simulink model "Acq_track"  (R2019b)
settings: Solver=VariableStepAuto  StartTime=0.0  StopTime=1  FixedStep=1/fs  RelTol=1e-3  EnableMultiTasking=on
values from neighbouring files (symbols this model uses):
  freq_vector = 2*pi*[(fc - 10e3):1e3:(fc+10e3)]    [config.m]
  fs = 16367600    [config.m]    (also in trackingCode.m)
  Len = ceil(ms*fs/1000)    [config.m]    (also in trackingCode.m = ceil((codeLength - remCodePhase)/(ca_freq/fs)))
  switch_time = 8*Len/fs    [config.m]
libraries: dspsigops x7, commfilt2 x6, dspstat3 x2, commseqgen3 x2, dspsrcs4 x1, simulink x1, simulink_extras x1
settings Model: Creator=nishantmittal  LastModifiedBy=sanke
settings SolverCC: AutoInsertRateTranBlk=on
settings OptimizationCC: DefaultUnderspecifiedDataType=single
settings DebuggingCC: ParameterPrecisionLossMsg=none

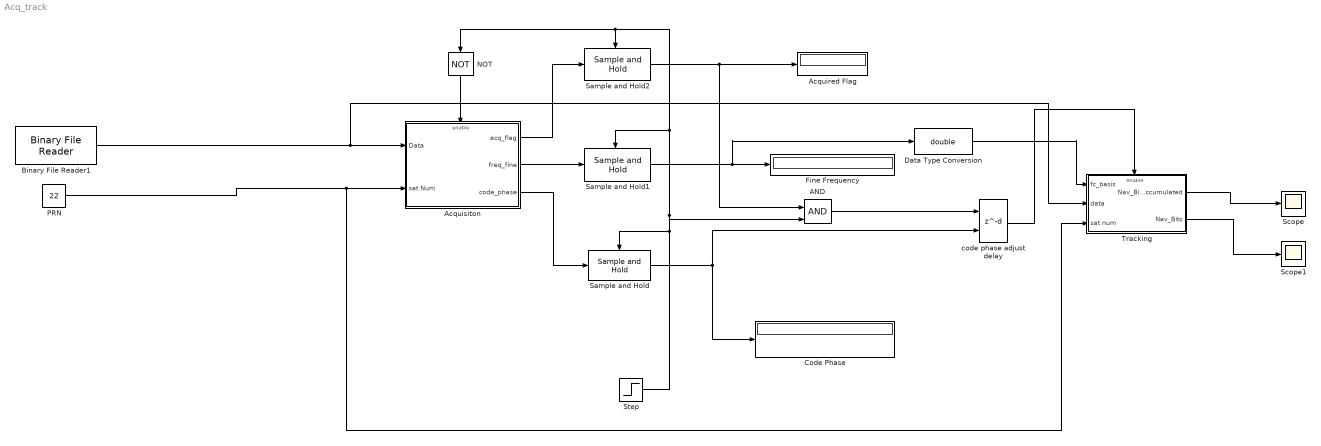
== system Acq_track ==
  AND : Logic  IconShape=distinctive  AllPortsSameDT=off  OutDataTypeStr=boolean
  Acquired Flag : Display
  Acquisiton : Subsystem
  Binary File Reader1 : dspsrcs4/Binary File Reader  Filename=/Users/nishantmittal/Documents/SURP/data/Acqisition/test/gioveAandB_short.bin  HeaderStructure=struct([])  DataType=int8  SamplesPerFrame=1  IsDataComplex=off  NumChannels=1  OutputEOF=off  SampleTime=1/fs  SimulateUsing=Code generation
      settings: SourceProductBaseCode=DS
  Code Phase : Display
  Data Type Conversion : DataTypeConversion  OutDataTypeStr=double
  Fine Frequency : Display
  NOT : Logic  Operator=NOT  IconShape=distinctive  AllPortsSameDT=off  OutDataTypeStr=boolean
  "PRN " : Constant  Value=22  OutDataTypeStr=single
  Sample and Hold : dspsigops/Sample and Hold  trig=Rising edge  initCond=0  latchinput=off
  Sample and Hold1 : dspsigops/Sample and Hold  trig=Rising edge  initCond=0  latchinput=off
  Sample and Hold2 : dspsigops/Sample and Hold  trig=Rising edge  initCond=0  latchinput=off
  Scope : Scope
  Scope1 : Scope
  Step : Step  Time=switch_time  SampleTime=1/fs
  Tracking : Subsystem
  code phase adjust delay : Delay  DelayLengthSource=Input port  DelayLength=1  DelayLengthUpperLimit=Len  InitialCondition=0  SampleTime=1/fs
      settings: InputPortMap=u0,p1
  wires:
  Binary File Reader1/1 -> Tracking/2(data), Acquisiton/1(Data)
  "PRN "/1 -> Tracking/3(sat num), Acquisiton/2(sat Num)
  Acquisiton/3(code_phase) -> Sample and Hold/1
  Sample and Hold/1 -> Code Phase/1, code phase adjust delay/2
  Acquisiton/2(freq_fine) -> Sample and Hold1/1
  Acquisiton/1(acq_flag) -> Sample and Hold2/1
  Step/1 -> AND/2, NOT/1, Sample and Hold2/Trigger, Sample and Hold1/Trigger, Sample and Hold/Trigger
  Tracking/1(Nav_Bits_Accumulated) -> Scope/1
  Sample and Hold1/1 -> Data Type Conversion/1, Fine Frequency/1
  AND/1 -> code phase adjust delay/1
  Sample and Hold2/1 -> AND/1, Acquired Flag/1
  NOT/1 -> Acquisiton/Enable
  code phase adjust delay/1 -> Tracking/Enable
  Data Type Conversion/1 -> Tracking/1(fc_basis)
  Tracking/2(Nav_Bits) -> Scope1/1

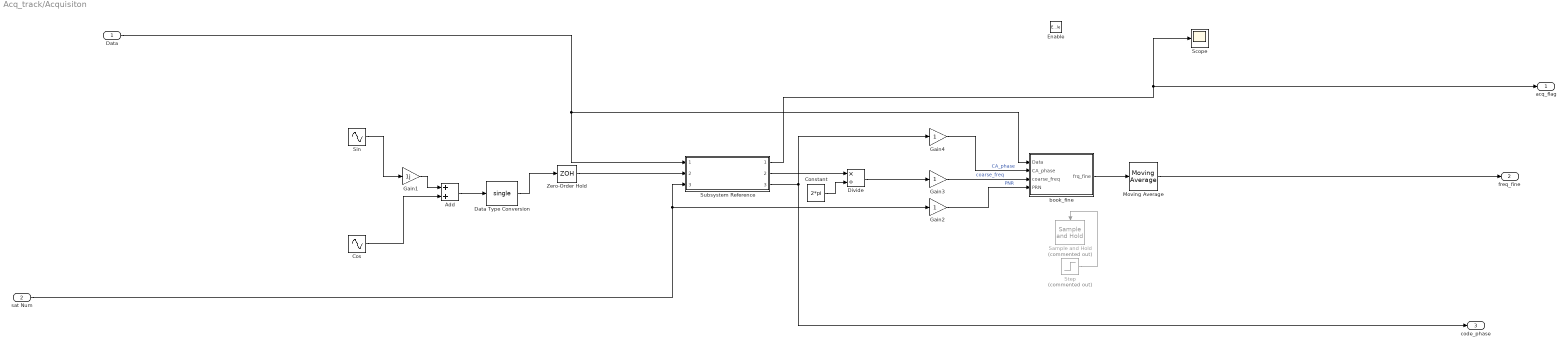
== system Acq_track/Acquisiton ==
  Data : Inport
  sat Num : Inport  Port=2
  Enable : EnablePort
  Add : Sum
  Constant : Constant  Value=2*pi  OutDataTypeStr=single
  Cos : Sin  Frequency=freq_vector  Phase=pi/2  SampleTime=1/fs
  Data Type Conversion : DataTypeConversion  OutDataTypeStr=single
  Divide : Product  Inputs=*/
  Gain1 : Gain  Gain=1j
  Gain2 : Gain
  Gain3 : Gain
  Gain4 : Gain  OutDataTypeStr=single
  Moving Average : dspstat3/Moving Average  Method=Sliding window  ForgettingFactorPort=off  SpecifyWindowLength=on  WindowLength=4  ForgettingFactor=0.9  SimulateUsing=Code generation
  Sample and Hold : dspsigops/Sample and Hold  Commented=on  trig=Rising edge  initCond=0  latchinput=off
  Scope : Scope
  "Sin " : Sin  Frequency=freq_vector  SampleTime=1/fs
  Step : Step  Commented=on  Time=0.00101  SampleTime=0
  Subsystem Reference : Subsystem  ReferencedSubsystem=acq_PNR
      settings: MinAlgLoopOccurrences=on
  Zero-Order Hold : ZeroOrderHold  SampleTime=1/fs
  book_fine : Subsystem
  acq_flag : Outport
  freq_fine : Outport  Port=2
  code_phase : Outport  Port=3
  wires:
  Moving Average/1 -> freq_fine/1
  Gain2/1 -> book_fine/4(PRN)  "PNR"
  Gain1/1 -> Add/1
  Subsystem Reference/2 -> Divide/1
  Data/1 -> book_fine/1(Data), Subsystem Reference/1
  Data Type Conversion/1 -> Zero-Order Hold/1
  "Sin "/1 -> Gain1/1
  Step/1 -> Sample and Hold/Trigger
  Gain4/1 -> book_fine/2(CA_phase)  "CA_phase"
  Add/1 -> Data Type Conversion/1
  Constant/1 -> Divide/2
  Cos/1 -> Add/2
  Gain3/1 -> book_fine/3(coarse_freq)  "coarse_freq"
  Subsystem Reference/1 -> acq_flag/1, Scope/1
  Divide/1 -> Gain3/1
  sat Num/1 -> Subsystem Reference/3, Gain2/1
  book_fine/1(frq_fine) -> Moving Average/1
  Zero-Order Hold/1 -> Subsystem Reference/2
  Subsystem Reference/3 -> code_phase/1, Gain4/1

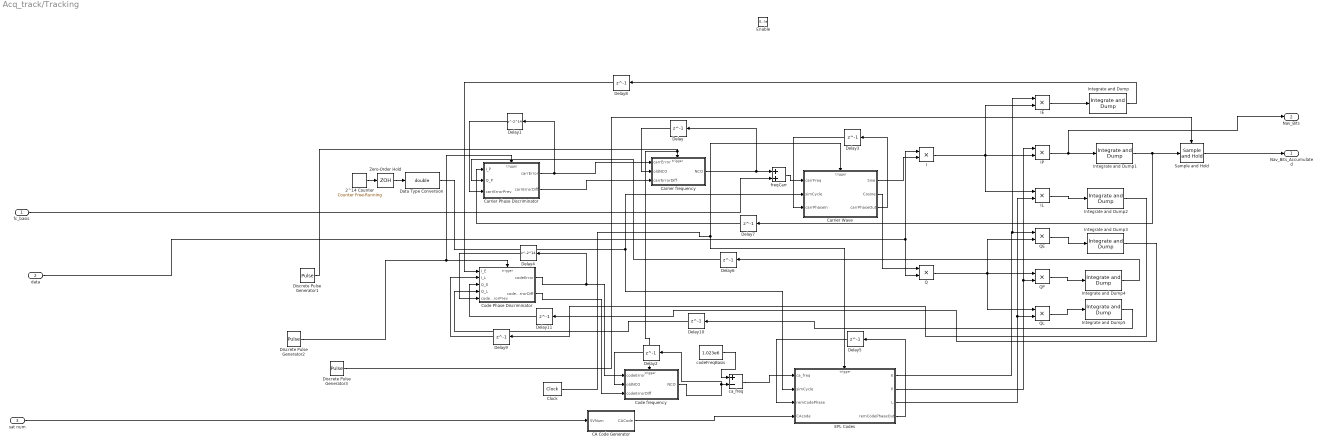
== system Acq_track/Tracking ==
  fc_basis : Inport
  data : Inport  Port=2
  sat num : Inport  Port=3
  Enable : EnablePort
  2^14 Counter : simulink/Sources/Counter Free-Running  NumBits=14  tsamp=1/fs
  CA Code Generator : Subsystem  TreatAsAtomicUnit=on
  Carrier Phase Discriminator : Subsystem  TreatAsAtomicUnit=on
  Carrier Wave : Subsystem  TreatAsAtomicUnit=on
  Carrier frequency : Subsystem  TreatAsAtomicUnit=on
  Clock : simulink_extras/Flip Flops/Clock  period=1/fs
  Code Phase Discriminator : Subsystem  TreatAsAtomicUnit=on
  Code frequency : Subsystem  TreatAsAtomicUnit=on
  Data Type Conversion : DataTypeConversion  OutDataTypeStr=double
  Delay{,2..3,5..11} (10 alike) : Delay  DelayLength=1  InitialCondition=0  SampleTime=1/fs
  Delay1 : Delay  DelayLength=2^14  InitialCondition=0  SampleTime=1/fs
  Delay4 : Delay  DelayLength=2^14  InitialCondition=0  SampleTime=1/fs
  Discrete Pulse Generator1 : DiscretePulseGenerator  Period=2^14  PulseWidth=5  PhaseDelay=2^14  SampleTime=1/fs
  Discrete Pulse Generator2 : DiscretePulseGenerator  Period=2^14  PulseWidth=5  PhaseDelay=2^14-20  SampleTime=1/fs
  Discrete Pulse Generator3 : DiscretePulseGenerator  Period=2^14  PulseWidth=5  PhaseDelay=2^14-2  SampleTime=1/fs
  EPL Codes : Subsystem  TreatAsAtomicUnit=on
  I : Product
  IE : Product
  IL : Product
  IP : Product
  Integrate and Dump{,1..5} (6 alike) : commfilt2/Integrate and Dump  obssamples=2^14  offsetsamples=0  nodump=on  roundingMode=Floor  overflowMode=off  outputDataTypeStr=Inherit: Same as accumulator  outputLastDataTypeStr=Inherit: Same as accumulator
  Q : Product
  QE : Product
  QL : Product
  QP : Product
  Sample and Hold : dspsigops/Sample and Hold  trig=Rising edge  initCond=0  latchinput=off
  Zero-Order Hold : ZeroOrderHold  SampleTime=1/fs
  ca_freq : Sum  Inputs=+-
  codeFreqBasis : Constant  Value=1.023e6
  freqCarr : Sum
  Nav_Bits_Accumulated : Outport
  Nav_Bits : Outport  Port=2
  wires:
  fc_basis/1 -> freqCarr/2
  Delay8/1 -> Code Phase Discriminator/1(I_E)
  Delay5/1 -> EPL Codes/3(remCodePhase)
  Delay6/1 -> Carrier Phase Discriminator/2(Q_P)
  Delay10/1 -> Code Phase Discriminator/4(Q_L)
  Delay11/1 -> Code Phase Discriminator/3(Q_E)
  sat num/1 -> CA Code Generator/1(SVNum)
  Integrate and Dump5/1 -> Delay10/1
  2^14 Counter/1 -> Zero-Order Hold/1
  Carrier Phase Discriminator/2(carrErrorDiff) -> Carrier frequency/3(carrErrorDiff)
  Integrate and Dump3/1 -> Delay11/1
  IE/1 -> Integrate and Dump/1
  ca_freq/1 -> EPL Codes/1(ca_freq)
  Carrier Wave/2(Cosine) -> Q/1
  Integrate and Dump4/1 -> Delay6/1
  EPL Codes/4(remCodePhaseOut) -> Delay5/1
  Q/1 -> QE/2, QL/1, QP/1
  Sample and Hold/1 -> Nav_Bits_Accumulated/1
  EPL Codes/2(P) -> IP/1, QP/2
  Delay7/1 -> Carrier Phase Discriminator/1(I_P)
  Carrier Wave/1(Sine) -> I/2
  Zero-Order Hold/1 -> Data Type Conversion/1
  Code Phase Discriminator/1(codeError) -> Delay4/1, Code frequency/1(codeError)
  Discrete Pulse Generator3/1 -> Sample and Hold/Trigger
  Delay2/1 -> Code frequency/2(oldNCO)
  EPL Codes/1(E) -> IE/1, QE/1
  QL/1 -> Integrate and Dump5/1
  codeFreqBasis/1 -> ca_freq/1
  Delay3/1 -> Carrier Wave/3(carrPhaseIn)
  IL/1 -> Integrate and Dump2/1
  Carrier Wave/3(carrPhaseOut) -> Delay3/1
  Integrate and Dump/1 -> Delay8/1
  Code Phase Discriminator/2(codeErrorDiff) -> Code frequency/3(codeErrorDiff)
  IP/1 -> Nav_Bits/1, Integrate and Dump1/1
  QE/1 -> Integrate and Dump3/1
  Discrete Pulse Generator2/1 -> Carrier Phase Discriminator/Trigger, Code Phase Discriminator/Trigger
  EPL Codes/3(L) -> IL/2, QL/2
  I/1 -> IL/1, IE/2, IP/2
  Data Type Conversion/1 -> Carrier Wave/2(simCycle), EPL Codes/2(simCycle)
  CA Code Generator/1(CACode) -> EPL Codes/4(CAcode)
  Integrate and Dump1/1 -> Delay7/1, Sample and Hold/1
  Carrier frequency/1(NCO) -> Delay/1, freqCarr/1
  Clock/1 -> EPL Codes/Trigger, Carrier Wave/Trigger
  freqCarr/1 -> Carrier Wave/1(carrFreq)
  Delay/1 -> Carrier frequency/2(oldNCO)
  Integrate and Dump2/1 -> Delay9/1
  data/1 -> Q/2, I/1
  Delay1/1 -> Carrier Phase Discriminator/3(carrErrorPrev)
  Delay4/1 -> Code Phase Discriminator/5(codeErrorPrev)
  Carrier Phase Discriminator/1(carrError) -> Carrier frequency/1(carrError), Delay1/1
  Discrete Pulse Generator1/1 -> Code frequency/Trigger, Carrier frequency/Trigger
  Code frequency/1(NCO) -> Delay2/1, ca_freq/2
  Delay9/1 -> Code Phase Discriminator/2(I_L)
  QP/1 -> Integrate and Dump4/1

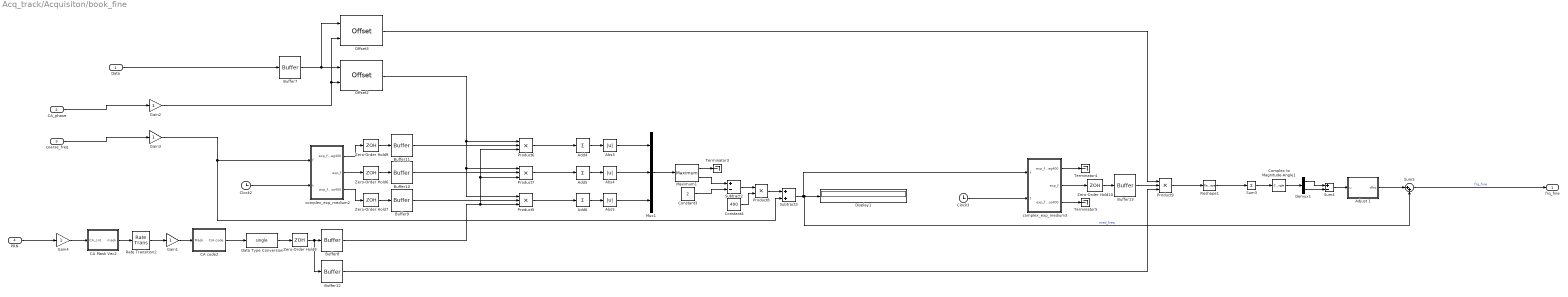
== system Acq_track/Acquisiton/book_fine ==
  Data : Inport
  CA_phase : Inport  Port=2
  coarse_freq : Inport  Port=3
  PRN : Inport  Port=4
  Abs3 : Abs
  Abs4 : Abs
  Abs5 : Abs
  Add4 : Sum  Inputs=+
  Add5 : Sum  Inputs=+
  Add6 : Sum  Inputs=+
  Adjust 1 : MATLAB Function  TreatAsAtomicUnit=on
  Buffer{8..11} (4 alike) : Buffer  N=Len  OutputFrames=off
  Buffer12 : Buffer  N=2*Len  OutputFrames=off
  Buffer13 : Buffer  N=2*Len  OutputFrames=off
  Buffer7 : Buffer  N=3*Len  OutputFrames=off
  CA Mask Vec2 : MATLAB Function  TreatAsAtomicUnit=on
  CA code2 : Subsystem
  Clock2 : Clock
  Clock3 : Clock
  Complex to Magnitude-Angle1 : ComplexToMagnitudeAngle  Output=Angle
  Constant3 : Constant  Value=2  OutDataTypeStr=single
  Constant4 : Constant  Value=400  OutDataTypeStr=single
  Data Type Conversion : DataTypeConversion  OutDataTypeStr=single
  Demux1 : Demux  Outputs=2
  Display1 : Display
  Gain1 : Gain  OutDataTypeStr=uint8
  Gain2 : Gain
  Gain3 : Gain
  Gain4 : Gain
  Maximum1 : dspstat3/Maximum  operation=maximum  fcn=Value and Index  indexBase=One  operateOver=Each column  Dimension=1  InputProcessing=Columns as channels (frame based)  reset=None  roiEnable=off  roiType=Rectangles  roiPortion=Entire ROI  roiOutput=Individual statistics for each ROI  roiFlag=off  roundingMode=Floor  overflowMode=off  accumDataTypeStr=Inherit: Same as product output  accumLastDataTypeStr=Inherit: Same as product output
  Mux1 : Mux  Inputs=3
  Offset2 : dspsigops/Offset  mode=Remove beginning samples  numDatOffPair=1  outWidthSpec=User-defined  outWidth=Len  actionOutRange=Clip
      settings: SourceProductBaseCode=DS
  Offset3 : dspsigops/Offset  mode=Remove beginning samples  numDatOffPair=1  outWidthSpec=User-defined  outWidth=2*Len  actionOutRange=Clip
      settings: SourceProductBaseCode=DS
  Product{5..7,9} (4 alike) : Product  Inputs=3
  Product8 : Product
  Rate Transition2 : RateTransition  Deterministic=off  OutPortSampleTime=1/(1.023e6)
  Reshape1 : Reshape  OutputDimensionality=Customize  OutputDimensions=[Len,2]
  Subtract2 : Sum  Inputs=+-
  Subtract3 : Sum
  Sum3 : Sum  Inputs=+  CollapseMode=Specified dimension
  Sum4 : Sum  Inputs=+-
  Sum5 : Sum  Inputs=|++
  Terminator3 : Terminator
  Terminator4 : Terminator
  Terminator5 : Terminator
  Zero-Order Hold{6..10} (5 alike) : ZeroOrderHold  SampleTime=1/fs
  complex_exp_medium2 : MATLAB Function  TreatAsAtomicUnit=on
  complex_exp_medium3 : MATLAB Function  TreatAsAtomicUnit=on
  frq_fine : Outport
  wires:
  Complex to Magnitude-Angle1/1 -> Demux1/1
  Add6/1 -> Abs5/1
  Clock2/1 -> complex_exp_medium2/2(t)
  Subtract3/1 -> complex_exp_medium3/1(f), Sum5/2, Display1/1  "med_freq"
  Product9/1 -> Reshape1/1
  Demux1/1 -> Sum4/1
  Constant3/1 -> Subtract2/2
  Buffer11/1 -> Product6/2
  Buffer13/1 -> Product9/2
  Abs5/1 -> Mux1/3
  Gain1/1 -> CA code2/1(Mask)
  Add4/1 -> Abs3/1
  Sum3/1 -> Complex to Magnitude-Angle1/1
  Clock3/1 -> complex_exp_medium3/2(t)
  Maximum1/1 -> Terminator3/1
  Constant4/1 -> Product8/2
  Demux1/2 -> Sum4/2
  Buffer8/1 -> Product6/3, Product7/3, Product5/3
  Offset3/1 -> Product9/1
  Buffer7/1 -> Offset3/1, Offset2/1
  complex_exp_medium3/2(exp_f) -> Zero-Order Hold10/1
  Add5/1 -> Abs4/1
  Product5/1 -> Add6/1
  Mux1/1 -> Maximum1/1
  Zero-Order Hold8/1 -> Buffer12/1, Buffer8/1
  Adjust 1/1(dfrq) -> Sum5/1
  Reshape1/1 -> Sum3/1
  complex_exp_medium2/2(exp_f) -> Zero-Order Hold6/1
  Buffer10/1 -> Product7/2
  Product8/1 -> Subtract3/1
  Buffer12/1 -> Product9/3
  Rate Transition2/1 -> Gain1/1
  Abs4/1 -> Mux1/2
  Buffer9/1 -> Product5/2
  Subtract2/1 -> Product8/1
  Zero-Order Hold9/1 -> Buffer11/1
  Product7/1 -> Add5/1
  complex_exp_medium2/3(exp_f_pos400) -> Zero-Order Hold7/1
  Sum4/1 -> Adjust 1/1(u)
  CA code2/1(C/A code) -> Data Type Conversion/1
  Zero-Order Hold7/1 -> Buffer9/1
  Product6/1 -> Add4/1
  Zero-Order Hold6/1 -> Buffer10/1
  CA Mask Vec2/1(mask) -> Rate Transition2/1
  Abs3/1 -> Mux1/1
  complex_exp_medium2/1(exp_f_neg400) -> Zero-Order Hold9/1
  complex_exp_medium3/3(exp_f_pos400) -> Terminator5/1
  Sum5/1 -> frq_fine/1  "frq_fine"
  complex_exp_medium3/1(exp_f_neg400) -> Terminator4/1
  Zero-Order Hold10/1 -> Buffer13/1
  Offset2/1 -> Product5/1, Product7/1, Product6/1
  Maximum1/2 -> Subtract2/1
  Gain2/1 -> Offset3/2, Offset2/2
  Gain3/1 -> Subtract3/2, complex_exp_medium2/1(f)
  Gain4/1 -> CA Mask Vec2/1(CA_cnt)
  PRN/1 -> Gain4/1
  coarse_freq/1 -> Gain3/1
  CA_phase/1 -> Gain2/1
  Data/1 -> Buffer7/1
  Data Type Conversion/1 -> Zero-Order Hold8/1

== system Acq_track/Tracking/CA Code Generator ==
  SVNum : Inport
  MATLAB Function : MATLAB Function  TreatAsAtomicUnit=on
  CACode : Outport
  wires:
  SVNum/1 -> MATLAB Function/1(svnum)
  MATLAB Function/1(y) -> CACode/1

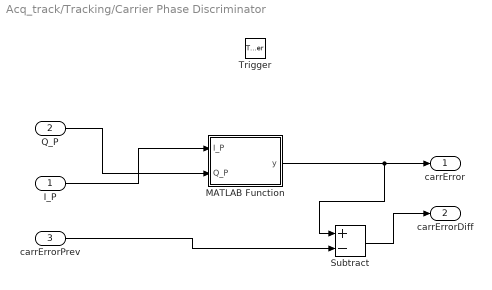
== system Acq_track/Tracking/Carrier Phase Discriminator ==
  I_P : Inport
  Q_P : Inport  Port=2
  carrErrorPrev : Inport  Port=3
  Trigger : TriggerPort  VariantControl=Variant  InitialTriggerSignalState=zero
  MATLAB Function : MATLAB Function  TreatAsAtomicUnit=on
  Subtract : Sum  Inputs=+-
  carrError : Outport  InitialOutput=0
  carrErrorDiff : Outport  Port=2  InitialOutput=0
  wires:
  MATLAB Function/1(y) -> Subtract/1, carrError/1
  carrErrorPrev/1 -> Subtract/2
  Subtract/1 -> carrErrorDiff/1
  I_P/1 -> MATLAB Function/1(I_P)
  Q_P/1 -> MATLAB Function/2(Q_P)

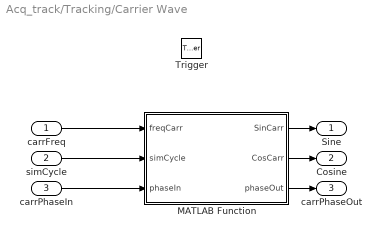
== system Acq_track/Tracking/Carrier Wave ==
  carrFreq : Inport
  simCycle : Inport  Port=2
  carrPhaseIn : Inport  Port=3
  Trigger : TriggerPort  VariantControl=Variant  InitialTriggerSignalState=zero
  MATLAB Function : MATLAB Function  TreatAsAtomicUnit=on
  Sine : Outport  InitialOutput=0
  Cosine : Outport  Port=2  InitialOutput=0
  carrPhaseOut : Outport  Port=3  InitialOutput=0
  wires:
  MATLAB Function/1(SinCarr) -> Sine/1
  carrFreq/1 -> MATLAB Function/1(freqCarr)
  simCycle/1 -> MATLAB Function/2(simCycle)
  carrPhaseIn/1 -> MATLAB Function/3(phaseIn)
  MATLAB Function/2(CosCarr) -> Cosine/1
  MATLAB Function/3(phaseOut) -> carrPhaseOut/1

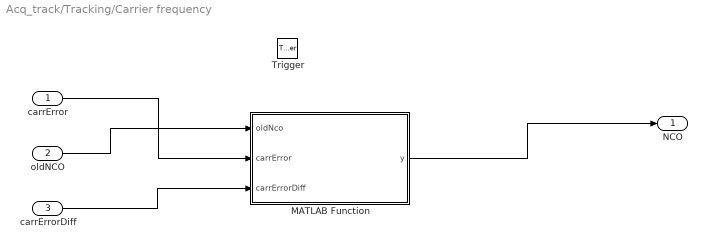
== system Acq_track/Tracking/Carrier frequency ==
  carrError : Inport
  oldNCO : Inport  Port=2
  carrErrorDiff : Inport  Port=3
  Trigger : TriggerPort  VariantControl=Variant  OutputDataType=double  InitialTriggerSignalState=zero
  MATLAB Function : MATLAB Function  TreatAsAtomicUnit=on
  NCO : Outport  InitialOutput=0
  wires:
  MATLAB Function/1(y) -> NCO/1
  carrError/1 -> MATLAB Function/2(carrError)
  oldNCO/1 -> MATLAB Function/1(oldNco)
  carrErrorDiff/1 -> MATLAB Function/3(carrErrorDiff)

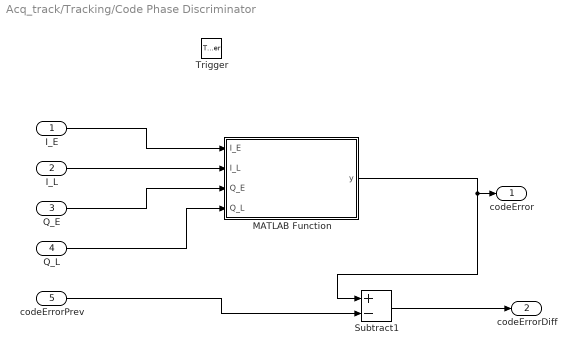
== system Acq_track/Tracking/Code Phase Discriminator ==
  I_E : Inport
  I_L : Inport  Port=2
  Q_E : Inport  Port=3
  Q_L : Inport  Port=4
  codeErrorPrev : Inport  Port=5
  Trigger : TriggerPort  VariantControl=Variant  InitialTriggerSignalState=zero
  MATLAB Function : MATLAB Function  TreatAsAtomicUnit=on
  Subtract1 : Sum  Inputs=+-
  codeError : Outport  InitialOutput=0
  codeErrorDiff : Outport  Port=2  InitialOutput=0
  wires:
  MATLAB Function/1(y) -> Subtract1/1, codeError/1
  codeErrorPrev/1 -> Subtract1/2
  Subtract1/1 -> codeErrorDiff/1
  I_E/1 -> MATLAB Function/1(I_E)
  I_L/1 -> MATLAB Function/2(I_L)
  Q_E/1 -> MATLAB Function/3(Q_E)
  Q_L/1 -> MATLAB Function/4(Q_L)

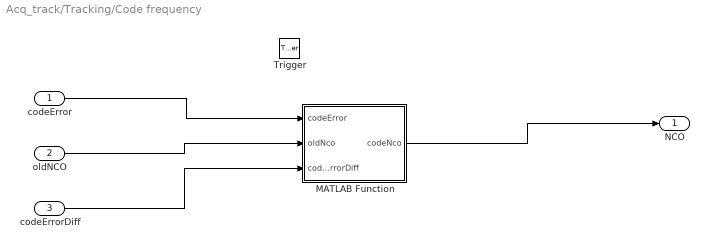
== system Acq_track/Tracking/Code frequency ==
  codeError : Inport
  oldNCO : Inport  Port=2
  codeErrorDiff : Inport  Port=3
  Trigger : TriggerPort  VariantControl=Variant  OutputDataType=double  InitialTriggerSignalState=zero
  MATLAB Function : MATLAB Function  TreatAsAtomicUnit=on
  NCO : Outport  InitialOutput=0
  wires:
  MATLAB Function/1(codeNco) -> NCO/1
  codeError/1 -> MATLAB Function/1(codeError)
  oldNCO/1 -> MATLAB Function/2(oldNco)
  codeErrorDiff/1 -> MATLAB Function/3(codeErrorDiff)

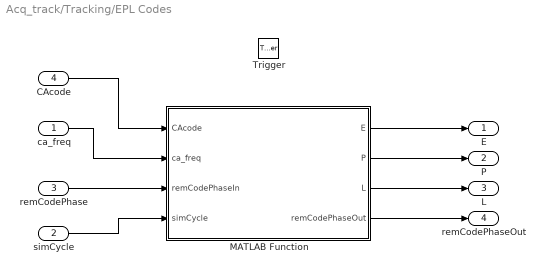
== system Acq_track/Tracking/EPL Codes ==
  ca_freq : Inport
  simCycle : Inport  Port=2
  remCodePhase : Inport  Port=3
  CAcode : Inport  Port=4
  Trigger : TriggerPort  VariantControl=Variant  InitialTriggerSignalState=zero
  MATLAB Function : MATLAB Function  TreatAsAtomicUnit=on
  E : Outport  InitialOutput=0
  P : Outport  Port=2  InitialOutput=0
  L : Outport  Port=3  InitialOutput=0
  remCodePhaseOut : Outport  Port=4  InitialOutput=0
  wires:
  CAcode/1 -> MATLAB Function/1(CAcode)
  ca_freq/1 -> MATLAB Function/2(ca_freq)
  remCodePhase/1 -> MATLAB Function/3(remCodePhaseIn)
  simCycle/1 -> MATLAB Function/4(simCycle)
  MATLAB Function/1(E) -> E/1
  MATLAB Function/2(P) -> P/1
  MATLAB Function/3(L) -> L/1
  MATLAB Function/4(remCodePhaseOut) -> remCodePhaseOut/1

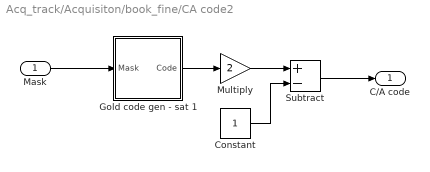
== system Acq_track/Acquisiton/book_fine/CA code2 ==
  Mask : Inport
  Constant : Constant
  Gold code gen - sat 1 : Subsystem
  Multiply : Gain  Gain=2
  Subtract : Sum  Inputs=+-
  C/A code : Outport
  wires:
  Subtract/1 -> C/A code/1
  Multiply/1 -> Subtract/1
  Gold code gen - sat 1/1(Code) -> Multiply/1
  Constant/1 -> Subtract/2
  Mask/1 -> Gold code gen - sat 1/1(Mask)

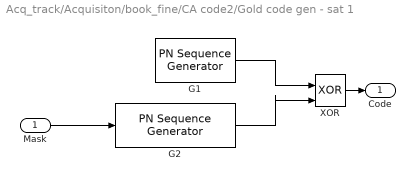
== system Acq_track/Acquisiton/book_fine/CA code2/Gold code gen - sat 1 ==
  Mask : Inport
  G1 : commseqgen3/PN Sequence Generator  poly=[10 7 0]  ini_sta=[1 1 1 1 1 1 1 1 1 1]  outBitMaskSource=Dialog parameter  shift=[0 0 0 0 0 0 0 0 0 1]  outVarSiz=off  maxOutSizeMode=Dialog parameter  maxOutSize=[10 1]  Ts=1/(1.023e6)  sampPerFrame=1  reset=off  bitPackedOutputs=off  outDataType=boolean  numPackedBits=8  bitPackDataSigned=off  bitPackedOutDType=double
  G2 : commseqgen3/PN Sequence Generator  poly=[10 8 7 4 2 1 0]  ini_sta=[1 1 1 1 1 1 1 1 1 1]  outBitMaskSource=Input port  shift=[0 1 0 0 0 1 0 0 0 0]  outVarSiz=off  maxOutSizeMode=Dialog parameter  maxOutSize=[10 1]  Ts=1/(1.023e6)  sampPerFrame=1  reset=off  bitPackedOutputs=off  outDataType=boolean  numPackedBits=8  bitPackDataSigned=off  bitPackedOutDType=double
  XOR : Logic  Operator=XOR  IconShape=distinctive  AllPortsSameDT=off  OutDataTypeStr=boolean
  Code : Outport
  wires:
  G2/1 -> XOR/2
  XOR/1 -> Code/1
  G1/1 -> XOR/1
  Mask/1 -> G2/1

== matlab function Acq_track/Acquisiton/book_fine/Adjust 1 ==
  data: u input; dfrq output
function dfrq = fcn(u)
u = u/(2*pi);
temp = u;
threshold = 0.23; 
if abs(u)>threshold% for angle adjustment 
    u = temp-1;
    if abs(u)>threshold
        u = temp+1; % end
        if abs(u)>0.22 % for pi phase shift correction
            u = temp-0.5;
            if abs(u)>threshold
                u = temp - 1.5;
                if abs(u)>threshold
                    u = temp+0.5;
                end
            end
        end
    end
end
dfrq = u*1000;

== matlab function Acq_track/Acquisiton/book_fine/CA Mask Vec2 ==
  data: CA_cnt input; mask output
function mask = fcn(CA_cnt)

phase = [2 6; 3 7; 4 8; 5 9; 1 9; 2 10; 1 8; 2 9; 3 10; 2 3; 3 4; 5 6; 6 7; 7 8; 8 9; 9 10; 1 4; 2 5; 3 6; 4 7; 5 8; 6 9; 1 3; 4 6; 5 7; 6 8; 7 9; 8 10; 1 6; 2 7; 3 8; 4 9];
mask_points = phase(CA_cnt, :);
mask = zeros(1,10);
mask(mask_points) = 1;

== matlab function Acq_track/Acquisiton/book_fine/complex_exp_medium2 ==
  data: exp_f_neg400 output; f input; exp_f output; t input; exp_f_pos400 output
function [exp_f_neg400, exp_f, exp_f_pos400] = fcn(f, t)
exp_f_neg400 = exp(1i*2*pi*(f-400)*t);
exp_f = exp(1i*2*pi*f*t);
exp_f_pos400 = exp(1i*2*pi*(f+400)*t);

== matlab function Acq_track/Acquisiton/book_fine/complex_exp_medium3 ==
  data: exp_f_neg400 output; f input; exp_f output; t input; exp_f_pos400 output
function [exp_f_neg400, exp_f, exp_f_pos400] = fcn(f, t)
exp_f_neg400 = exp(1i*2*pi*(f-400)*t);
exp_f = exp(1i*2*pi*f*t);
exp_f_pos400 = exp(1i*2*pi*(f+400)*t);

== matlab function Acq_track/Tracking/CA Code Generator/MATLAB Function ==
  data: svnum input; y output
function y = CAGen(svnum)
g2s = [5;6;7;8;17;18;139;140;141;251;252;254;255;256;257;258; 469;470;471; ...
     472;473;474;509;512;513;514;515;516;859;860;861;862]; 
 
g2shift = g2s(svnum,1);

% Generate G1 code
% load shift register 
reg = -1*ones(1,10);
g1 = zeros(1,1023);
for i = 1:1023
    g1(i) = reg(10);
    save1 = reg(3)*reg(10); 
    reg(1,2:10) = reg(1:1:9); 
    reg(1) = save1;
end

%  Generate G2 code 
% load shift register 
reg = -1*ones(1,10);
g2 = zeros(1,1023);
for i = 1:1023
    g2(i) = reg(10);
    save2 = reg(2)*reg(3)*reg(6)*reg(8)*reg(9)*reg(10);
    reg(1,2:10) = reg(1:1:9);
    reg(1) = save2; 
end

% Shift G2 code
g2tmp = zeros(1,1023);
g2tmp(1,1:g2shift) = g2(1,1023-g2shift+1:1023); 
g2tmp(1,g2shift+1:1023) = g2(1,1:1023-g2shift); 
g2 = g2tmp;
%
% Form single sample C/A code by multiplying G1 and G2 %
ss_ca = g1.*g2;
y = -ss_ca;

== matlab function Acq_track/Tracking/Carrier Phase Discriminator/MATLAB Function ==
  data: I_P input; y output; Q_P input
function y = carrError(I_P, Q_P)

if I_P~=0 || Q_P~= 0
    y = atan(Q_P / I_P) / (2.0 * pi);
else
    y=0;
end

== matlab function Acq_track/Tracking/Carrier Wave/MATLAB Function ==
  data: freqCarr input; SinCarr output; simCycle input; phaseIn input; CosCarr output; phaseOut output
function [SinCarr, CosCarr, phaseOut] = fcn(freqCarr, simCycle, phaseIn)

SinCarr = sin(freqCarr*2*pi*simCycle/16367600 + phaseIn);
CosCarr = cos(freqCarr*2*pi*simCycle/16367600 + phaseIn);
if simCycle < 2^14 - 1
    phaseOut = phaseIn;
else
    phaseOut = rem(freqCarr*2*pi*2^14/16367600+phaseIn, 2*pi);
end

== matlab function Acq_track/Tracking/Carrier frequency/MATLAB Function ==
  data: oldNco input; y output; carrError input; carrErrorDiff input
function y = carrNco(oldNco, carrError, carrErrorDiff)

tau1carr = 1.117551020408163e-04;
tau2carr = 0.0296;
PDIcarr = 0;

y = oldNco + (tau2carr/tau1carr) * (carrErrorDiff) + carrError * (PDIcarr/tau1carr);

== matlab function Acq_track/Tracking/Code Phase Discriminator/MATLAB Function ==
  data: I_E input; y output; I_L input; Q_E input; Q_L input
function y = codeError(I_E, I_L, Q_E, Q_L)


if I_E~=0 || I_L~=0 || Q_E~= 0 || Q_L ~= 0
    y = (sqrt(I_E * I_E + Q_E * Q_E) - sqrt(I_L * I_L + Q_L * Q_L)) / ...
                (sqrt(I_E * I_E + Q_E * Q_E) + sqrt(I_L * I_L + Q_L * Q_L));
else
    y=0;
end

== matlab function Acq_track/Tracking/Code frequency/MATLAB Function ==
  data: codeError input; codeNco output; oldNco input; codeErrorDiff input
function codeNco  = fcn(codeError, oldNco, codeErrorDiff)

tau1code = 0.011175510204082;
tau2code = 0.148;
PDIcode = 0;

codeNco = oldNco + (tau2code/tau1code) * (codeErrorDiff) + codeError * (PDIcode/tau1code);

== matlab function Acq_track/Tracking/EPL Codes/MATLAB Function ==
  data: CAcode input; E output; ca_freq input; remCodePhaseIn input; simCycle input; P output; L output; remCodePhaseOut output
function [E, P, L, remCodePhaseOut] = EPLGenerator(CAcode, ca_freq, remCodePhaseIn, simCycle)

CAcode = [CAcode(1023) CAcode CAcode];

%Early
tcode = ceil(remCodePhaseIn-0.5+simCycle*ca_freq/16367600)+1;
E = CAcode(tcode);

%Late
tcode = ceil(remCodePhaseIn+0.5+simCycle*ca_freq/16367600)+1;
L = CAcode(tcode);

%Prompt
tcode = ceil(remCodePhaseIn+simCycle*ca_freq/16367600)+1;
P = CAcode(tcode);

if simCycle < 2^14 - 1
    remCodePhaseOut = remCodePhaseIn;
else
    remCodePhaseOut = remCodePhaseIn+2^14*ca_freq/16367600 - 1023.0;
end
